simulink model "Кирхгоф"  (R2020b)
settings: Solver=FixedStepAuto  StartTime=0.0  StopTime=0.4  FixedStep=10e-5  RelTol=1e-3
libraries: powerlib x11
settings Model: Creator=New-life  LastModifiedBy=New-life

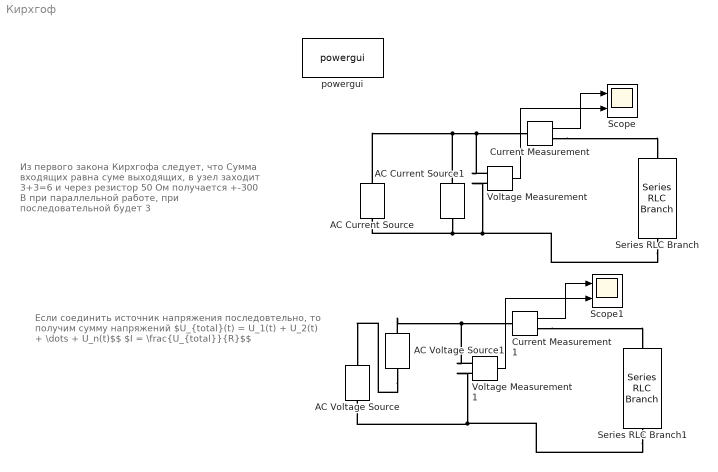
== system Кирхгоф ==
  note: Если соединить источник напряжения последовтельно,
      | то получим сумму напряжений
      | $U_{total}(t) = U_1(t) + U_2(t) + \dots + U_n(t)$$ $I = \frac{U_{total}}{R}$$
  note: Из первого закона Кирхгофа следует, что
      | Сумма входящих равна суме выходящих, в
      | узел заходит 3+3=6 и через резистор 50 Ом
      | получается +-300 В при параллельной работе,
      | при последовательной
      | будет 3
  AC Current Source : powerlib/Electrical Sources/AC Current Source  Amplitude=3  Phase=0  Frequency=50  SampleTime=0  Measurements=None
      settings: SourceProductBaseCode=PS
  AC Current Source1 : powerlib/Electrical Sources/AC Current Source  Amplitude=3  Phase=0  Frequency=50  SampleTime=0  Measurements=None
      settings: SourceProductBaseCode=PS
  AC Voltage Source : powerlib/Electrical Sources/AC Voltage Source  Amplitude=100  Phase=0  Frequency=60  SampleTime=0  Measurements=None  BusType=swing  Pref=10e3  Qref=0  Qmin=-inf  Qmax=+inf
  AC Voltage Source1 : powerlib/Electrical Sources/AC Voltage Source  Amplitude=100  Phase=0  Frequency=60  SampleTime=0  Measurements=None  BusType=swing  Pref=10e3  Qref=0  Qmin=-inf  Qmax=+inf
  Current Measurement : powerlib/Measurements/Current Measurement  PhasorSimulation=off  OutputType=Complex  PSBequivalent=0
  Current Measurement1 : powerlib/Measurements/Current Measurement  PhasorSimulation=off  OutputType=Complex  PSBequivalent=0
  Scope : Scope  NumInputPorts=2
  Scope1 : Scope  NumInputPorts=2
  Series RLC Branch : powerlib/Elements/Series RLC Branch  LConnTagsString=__new0  RConnTagsString=__new0  BranchType=R  Resistance=50  Inductance=1e-3  SetiL0=off  InitialCurrent=0  Capacitance=1e-6  Setx0=off  InitialVoltage=0  Measurements=None
  Series RLC Branch1 : powerlib/Elements/Series RLC Branch  LConnTagsString=__new0  RConnTagsString=__new0  BranchType=R  Resistance=50  Inductance=1e-3  SetiL0=off  InitialCurrent=0  Capacitance=1e-6  Setx0=off  InitialVoltage=0  Measurements=None
  Voltage Measurement : powerlib/Measurements/Voltage Measurement  PhasorSimulation=off  OutputType=Complex  PSBequivalent=0
  Voltage Measurement1 : powerlib/Measurements/Voltage Measurement  PhasorSimulation=off  OutputType=Complex  PSBequivalent=0
  powergui : powerlib/powergui  Priority=1  SimulationMode=Continuous  SampleTime=50e-6  frequency=60  Iterations=50  frequencyindice=60  Pbase=100e6  ErrMax=1e-4  UnitsV=kV  UnitsW=MW  buscounter=0  FunctionMessages=off  echomessages=off  EnableUseOfTLC=off  CurrentSourceSwitches=off  DisableSnubberDevices=off  DisableRonSwitches=off  DisableVfSwitches=off  DisplayEquations=off  AutomaticDiscreteSolvers=off  SolverType=Tustin/Backward Euler (TBE)  Interpol=off  ExternalGateDelay=off  methode=off  Ts=100  x0status=blocks  SPID=on  SwTol=0  HookPort=off  NonlinearTolerance=1e-4  nMaxIteration=100  ContinueOnMaxIteration=off  RestoreLinks=warning  ResistiveCurrentMeasurement=off  Frange=[0:2:500]  Ylog=off  Xlog=on  ShowGrid=off  save=off  variable=ZData  structure=0  ZoomFFT=off  StartTime=0.0  cycles=1  DisplayStyle=1  fundamental=60  FreqAxis=off  MaxFrequency=1000  frequencyindicesteady=1  RmsSteady=1  display=off
  wires:
  Current Measurement/1 -> Scope/1
  Voltage Measurement/1 -> Scope/2
  Voltage Measurement1/1 -> Scope1/2
  Current Measurement1/1 -> Scope1/1
  connections:
  AC Current Source/RConn1 -- AC Current Source1/RConn1 -- Voltage Measurement/LConn1 -- Current Measurement/LConn1
  Series RLC Branch/RConn1 -- Voltage Measurement/LConn2 -- AC Current Source1/LConn1 -- AC Current Source/LConn1
  Current Measurement/RConn1 -- Series RLC Branch/LConn1
  AC Voltage Source1/RConn1 -- AC Voltage Source/LConn1
  Voltage Measurement1/LConn2 -- Series RLC Branch1/RConn1 -- AC Voltage Source/RConn1
  Current Measurement1/RConn1 -- Series RLC Branch1/LConn1
  Voltage Measurement1/LConn1 -- AC Voltage Source1/LConn1 -- Current Measurement1/LConn1
